simulink model "IMfault"  (R2017a)
settings: Solver=FixedStepAuto  StartTime=0.0  StopTime=0.6  MaxStep=1e-4  RelTol=1e-3
libraries: powerlib x24, dspxfrm3 x3, dspspect3 x3
settings Model: Creator=saeed  LastModifiedBy=Lenovo

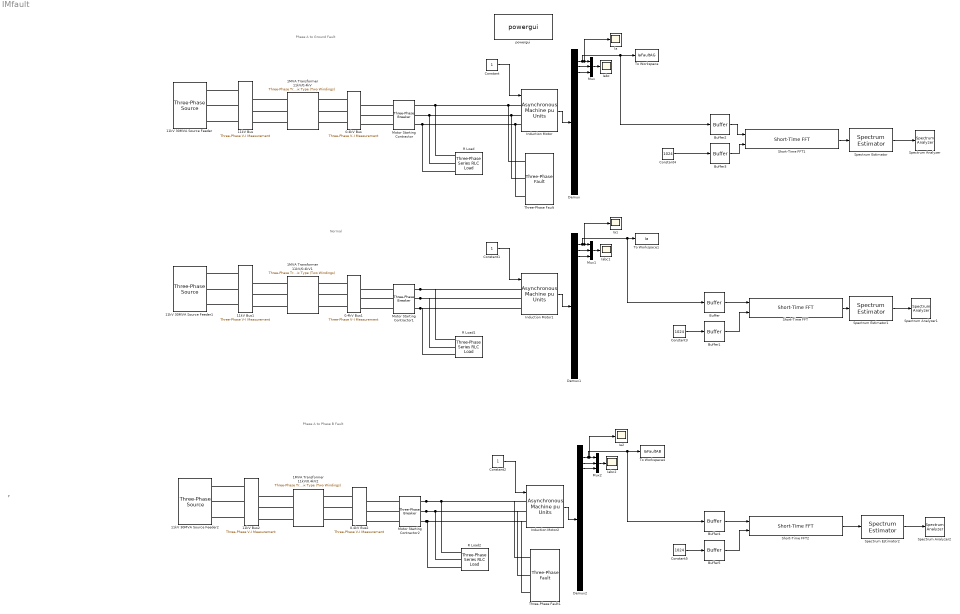
== system IMfault ==
  note: Normal
  note: P
  note: Phase A to Ground
      | Fault
  note: Phase A to Phase B
      | Fault
  0.4kV Bus : powerlib/Measurements/Three-Phase V-I Measurement  VoltageMeasurement=no  SetLabelV=off  LabelV=Vabc  Vpu=off  VpuLL=off  CurrentMeasurement=yes  SetLabelI=off  LabelI=Iabc  Ipu=off  Pbase=100e6  Vbase=500e3  OutputType=Complex  PhasorSimulation=off  PSBequivalent=0
  0.4kV Bus1 : powerlib/Measurements/Three-Phase V-I Measurement  VoltageMeasurement=no  SetLabelV=off  LabelV=Vabc  Vpu=off  VpuLL=off  CurrentMeasurement=yes  SetLabelI=off  LabelI=Iabc  Ipu=off  Pbase=100e6  Vbase=500e3  OutputType=Complex  PhasorSimulation=off  PSBequivalent=0
  0.4kV Bus2 : powerlib/Measurements/Three-Phase V-I Measurement  VoltageMeasurement=no  SetLabelV=off  LabelV=Vabc  Vpu=off  VpuLL=off  CurrentMeasurement=yes  SetLabelI=off  LabelI=Iabc  Ipu=off  Pbase=100e6  Vbase=500e3  OutputType=Complex  PhasorSimulation=off  PSBequivalent=0
  11kV Bus : powerlib/Measurements/Three-Phase V-I Measurement  VoltageMeasurement=no  SetLabelV=off  LabelV=Vabc  Vpu=off  VpuLL=off  CurrentMeasurement=yes  SetLabelI=off  LabelI=Iabc  Ipu=off  Pbase=100e6  Vbase=500e3  OutputType=Complex  PhasorSimulation=off  PSBequivalent=0
  11kV Bus1 : powerlib/Measurements/Three-Phase V-I Measurement  VoltageMeasurement=no  SetLabelV=off  LabelV=Vabc  Vpu=off  VpuLL=off  CurrentMeasurement=yes  SetLabelI=off  LabelI=Iabc  Ipu=off  Pbase=100e6  Vbase=500e3  OutputType=Complex  PhasorSimulation=off  PSBequivalent=0
  11kV Bus2 : powerlib/Measurements/Three-Phase V-I Measurement  VoltageMeasurement=no  SetLabelV=off  LabelV=Vabc  Vpu=off  VpuLL=off  CurrentMeasurement=yes  SetLabelI=off  LabelI=Iabc  Ipu=off  Pbase=100e6  Vbase=500e3  OutputType=Complex  PhasorSimulation=off  PSBequivalent=0
  11kV 30MVA Source Feeder : powerlib/Electrical Sources/Three-Phase Source  InternalConnection=Yg  VoltagePhases=off  Voltage=25e3  PhaseAngle=0  Voltage_phases=[25e3 25e3 25e3]/sqrt(3)  PhaseAngles_phases=[0 -120 +120]  Frequency=50  NonIdealSource=on  SpecifyImpedance=off  Resistance=0.8929  Inductance=16.58e-3  ShortCircuitLevel=100e6  BaseVoltage=25e3  XRratio=7  BusType=swing  Pref=10e3  Qref=0  Prefabc=[10e3, 10e3, 10e3]  Qrefabc=[0, 0, 0]  Qmin=-inf  Qmax=inf
  11kV 30MVA Source Feeder1 : powerlib/Electrical Sources/Three-Phase Source  InternalConnection=Yg  VoltagePhases=off  Voltage=25e3  PhaseAngle=0  Voltage_phases=[25e3 25e3 25e3]/sqrt(3)  PhaseAngles_phases=[0 -120 +120]  Frequency=50  NonIdealSource=on  SpecifyImpedance=off  Resistance=0.8929  Inductance=16.58e-3  ShortCircuitLevel=100e6  BaseVoltage=25e3  XRratio=7  BusType=swing  Pref=10e3  Qref=0  Prefabc=[10e3, 10e3, 10e3]  Qrefabc=[0, 0, 0]  Qmin=-inf  Qmax=inf
  11kV 30MVA Source Feeder2 : powerlib/Electrical Sources/Three-Phase Source  InternalConnection=Yg  VoltagePhases=off  Voltage=25e3  PhaseAngle=0  Voltage_phases=[25e3 25e3 25e3]/sqrt(3)  PhaseAngles_phases=[0 -120 +120]  Frequency=50  NonIdealSource=on  SpecifyImpedance=off  Resistance=0.8929  Inductance=16.58e-3  ShortCircuitLevel=100e6  BaseVoltage=25e3  XRratio=7  BusType=swing  Pref=10e3  Qref=0  Prefabc=[10e3, 10e3, 10e3]  Qrefabc=[0, 0, 0]  Qmin=-inf  Qmax=inf
  1MVA Transformer 11kV/0.4kV : powerlib/Elements/Three-Phase Transformer Inductance Matrix Type (Two Windings)  CoreType=Three-limb or five-limb core  Winding1Connection=Yg  Winding2Connection=Yg  AutoTransformer=on  Measurements=None  NominalPower=[100e3, 50]  VLLnom=[2400, 600]  WindingResistances=[0.01, 0.01]  NoLoadIexcPos=2  NoLoadPlossPos=1000  ShortCircuitReactancePos=0.06  ShortCircuitReactancePosAuto=0.06  NoLoadIexcZero=100  NoLoadPlossZero=1500  ShortCircuitReactanceZero=0.03  ShortCircuitReactanceZeroAuto=0.03
      settings: SourceProductName=Simscape Power Systems  SourceProductBaseCode=PS
  1MVA Transformer 11kV/0.4kV1 : powerlib/Elements/Three-Phase Transformer Inductance Matrix Type (Two Windings)  CoreType=Three-limb or five-limb core  Winding1Connection=Yg  Winding2Connection=Yg  AutoTransformer=on  Measurements=None  NominalPower=[100e3, 50]  VLLnom=[2400, 600]  WindingResistances=[0.01, 0.01]  NoLoadIexcPos=2  NoLoadPlossPos=1000  ShortCircuitReactancePos=0.06  ShortCircuitReactancePosAuto=0.06  NoLoadIexcZero=100  NoLoadPlossZero=1500  ShortCircuitReactanceZero=0.03  ShortCircuitReactanceZeroAuto=0.03
      settings: SourceProductName=Simscape Power Systems  SourceProductBaseCode=PS
  1MVA Transformer 11kV/0.4kV2 : powerlib/Elements/Three-Phase Transformer Inductance Matrix Type (Two Windings)  CoreType=Three-limb or five-limb core  Winding1Connection=Yg  Winding2Connection=Yg  AutoTransformer=on  Measurements=None  NominalPower=[100e3, 50]  VLLnom=[2400, 600]  WindingResistances=[0.01, 0.01]  NoLoadIexcPos=2  NoLoadPlossPos=1000  ShortCircuitReactancePos=0.06  ShortCircuitReactancePosAuto=0.06  NoLoadIexcZero=100  NoLoadPlossZero=1500  ShortCircuitReactanceZero=0.03  ShortCircuitReactanceZeroAuto=0.03
      settings: SourceProductName=Simscape Power Systems  SourceProductBaseCode=PS
  Buffer{,1..5} (6 alike) : Buffer  N=512  OutputFrames=off
  Constant : Constant
  Constant1 : Constant
  Constant2 : Constant
  Constant3 : Constant  Value=1024
  Constant4 : Constant  Value=1024
  Constant5 : Constant  Value=1024
  Demux : Demux  Outputs=22
  Demux1 : Demux  Outputs=22
  Demux2 : Demux  Outputs=22
  Ia : Scope
  Ia1 : Scope
  Ia2 : Scope
  Iabc : Scope
  Iabc1 : Scope
  Iabc2 : Scope
  Induction Motor : powerlib/Machines/Asynchronous Machine pu Units  RotorType=Squirrel-cage  PresetModel=No  MechanicalLoad=Speed w  ShowDetailedParameters=on  ReferenceFrame=Rotor  Units=pu  MeasurementBus=on  NominalParameters=[3730 460 50]  Stator=[0.01965 0.0397]  Rotor=[0.01909 0.0397]  Cage1=[0.01909 0.0397]  Cage2=[0.01909 0.0397]  Lm=1.354  Mechanical=[0.09526 0.05479 2]  PolePairs=2  InitialConditions="[ 1,0   0,0,0   0,0,0 ]"  SimulateSaturation=off  Saturation="[0.212,0.4201,0.8125,1.0979,1.4799,2.2457,3.2586,4.5763,6.4763 ;   0.5,0.7,0.9,1,1.1,1.2 ,1.3,1.4,1.5]"  LoadFlowParameters=0  TsPowergui=0  TsBlock=-1  IterativeModel=Trapezoidal non iterative  IterativeDiscreteModel=Trapezoidal non iterative  Pmec=0
      settings: SourceProductName=Simscape Power Systems  SourceProductBaseCode=PS
  Induction Motor1 : powerlib/Machines/Asynchronous Machine pu Units  RotorType=Squirrel-cage  PresetModel=No  MechanicalLoad=Speed w  ShowDetailedParameters=on  ReferenceFrame=Rotor  Units=pu  MeasurementBus=on  NominalParameters=[3730 460 50]  Stator=[0.01965 0.0397]  Rotor=[0.01909 0.0397]  Cage1=[0.01909 0.0397]  Cage2=[0.01909 0.0397]  Lm=1.354  Mechanical=[0.09526 0.05479 2]  PolePairs=2  InitialConditions="[ 1,0   0,0,0   0,0,0 ]"  SimulateSaturation=off  Saturation="[0.212,0.4201,0.8125,1.0979,1.4799,2.2457,3.2586,4.5763,6.4763 ;   0.5,0.7,0.9,1,1.1,1.2 ,1.3,1.4,1.5]"  LoadFlowParameters=0  TsPowergui=0  TsBlock=-1  IterativeModel=Trapezoidal non iterative  IterativeDiscreteModel=Trapezoidal non iterative  Pmec=0
      settings: SourceProductName=Simscape Power Systems  SourceProductBaseCode=PS
  Induction Motor2 : powerlib/Machines/Asynchronous Machine pu Units  RotorType=Squirrel-cage  PresetModel=No  MechanicalLoad=Speed w  ShowDetailedParameters=on  ReferenceFrame=Rotor  Units=pu  MeasurementBus=on  NominalParameters=[3730 460 50]  Stator=[0.01965 0.0397]  Rotor=[0.01909 0.0397]  Cage1=[0.01909 0.0397]  Cage2=[0.01909 0.0397]  Lm=1.354  Mechanical=[0.09526 0.05479 2]  PolePairs=2  InitialConditions="[ 1,0   0,0,0   0,0,0 ]"  SimulateSaturation=off  Saturation="[0.212,0.4201,0.8125,1.0979,1.4799,2.2457,3.2586,4.5763,6.4763 ;   0.5,0.7,0.9,1,1.1,1.2 ,1.3,1.4,1.5]"  LoadFlowParameters=0  TsPowergui=0  TsBlock=-1  IterativeModel=Trapezoidal non iterative  IterativeDiscreteModel=Trapezoidal non iterative  Pmec=0
      settings: SourceProductName=Simscape Power Systems  SourceProductBaseCode=PS
  Motor Starting Contractor : powerlib/Elements/Three-Phase Breaker  InitialState=open  SwitchA=on  SwitchB=on  SwitchC=on  SwitchTimes=[0.005]  External=off  BreakerResistance=0.01  SnubberResistance=1e6  SnubberCapacitance=inf  Measurements=None
  Motor Starting Contractor1 : powerlib/Elements/Three-Phase Breaker  InitialState=open  SwitchA=on  SwitchB=on  SwitchC=on  SwitchTimes=[0.005]  External=off  BreakerResistance=0.01  SnubberResistance=1e6  SnubberCapacitance=inf  Measurements=None
  Motor Starting Contractor2 : powerlib/Elements/Three-Phase Breaker  InitialState=open  SwitchA=on  SwitchB=on  SwitchC=on  SwitchTimes=[0.005]  External=off  BreakerResistance=0.01  SnubberResistance=1e6  SnubberCapacitance=inf  Measurements=None
  Mux : Mux  Inputs=3
  Mux1 : Mux  Inputs=3
  Mux2 : Mux  Inputs=3
  R Load : powerlib/Elements/Three-Phase Series RLC Load  LConnTagsString=A|B|C  Configuration=Y (grounded)  NominalVoltage=1000  Vabc=[1e3 1e3 1e3]  Vabcp=[1e3 1e3 1e3]  NominalFrequency=50  UnbalancedPower=off  ActivePower=10e3  InductivePower=100  CapacitivePower=100  Pabc=[10e3 9e3 11e3]  QLabc=[100 90 110]  QCabc=[100 90 110]  Pabcp=[10e3 9e3 11e3]  QLabcp=[100 90 110]  QCabcp=[100 90 110]  Measurements=None  LoadType=constant I
  R Load1 : powerlib/Elements/Three-Phase Series RLC Load  LConnTagsString=A|B|C  Configuration=Y (grounded)  NominalVoltage=1000  Vabc=[1e3 1e3 1e3]  Vabcp=[1e3 1e3 1e3]  NominalFrequency=60  UnbalancedPower=off  ActivePower=10e3  InductivePower=100  CapacitivePower=100  Pabc=[10e3 9e3 11e3]  QLabc=[100 90 110]  QCabc=[100 90 110]  Pabcp=[10e3 9e3 11e3]  QLabcp=[100 90 110]  QCabcp=[100 90 110]  Measurements=None  LoadType=constant I
  R Load2 : powerlib/Elements/Three-Phase Series RLC Load  LConnTagsString=A|B|C  Configuration=Y (grounded)  NominalVoltage=1000  Vabc=[1e3 1e3 1e3]  Vabcp=[1e3 1e3 1e3]  NominalFrequency=50  UnbalancedPower=off  ActivePower=10e3  InductivePower=100  CapacitivePower=100  Pabc=[10e3 9e3 11e3]  QLabc=[100 90 110]  QCabc=[100 90 110]  Pabcp=[10e3 9e3 11e3]  QLabcp=[100 90 110]  QCabcp=[100 90 110]  Measurements=None  LoadType=constant I
  Short-Time FFT : dspxfrm3/Short-Time FFT  W=512  OvLap=256  M=1024
      settings: SourceProductName=DSP System Toolbox  SourceProductBaseCode=DS
  Short-Time FFT1 : dspxfrm3/Short-Time FFT  W=512  OvLap=216  M=1024
      settings: SourceProductName=DSP System Toolbox  SourceProductBaseCode=DS
  Short-Time FFT2 : dspxfrm3/Short-Time FFT  W=512  OvLap=256  M=1024
      settings: SourceProductName=DSP System Toolbox  SourceProductBaseCode=DS
  Spectrum Analyzer : SpectrumAnalyzer
  Spectrum Analyzer1 : SpectrumAnalyzer
  Spectrum Analyzer2 : SpectrumAnalyzer
  Spectrum Estimator : dspspect3/Spectrum Estimator  Method=Filter bank  NumTapsPerBand=12  SpectrumType=Power density  FrequencyResolutionMethod=Auto  FilterBankResolutionMethod=Auto  RBW=5  WindowLength=1024  FrequencyBandsSource=Same as input frame size  FrequencyBands=1024  FFTLengthSource=Auto  FFTLength=1024  InheritSampleRate=on  SampleRate=44100  Window=Hann  SidelobeAttenuation=60  SpectralAverages=1  Overlap=0  ReferenceLoad=1  FrequencyRange=Centered  PowerUnits=dBm  OutputMaxHoldSpectrum=off  OutputMinHoldSpectrum=off  OutputFrequencyVector=off  OutputRBW=off  SimulateUsing=Code generation
      settings: SourceProductName=DSP System Toolbox  SourceProductBaseCode=DS
  Spectrum Estimator1 : dspspect3/Spectrum Estimator  Method=Filter bank  NumTapsPerBand=12  SpectrumType=Power  FrequencyResolutionMethod=Auto  FilterBankResolutionMethod=Auto  RBW=5  WindowLength=1024  FrequencyBandsSource=Same as input frame size  FrequencyBands=1024  FFTLengthSource=Auto  FFTLength=1024  InheritSampleRate=on  SampleRate=44100  Window=Hann  SidelobeAttenuation=60  SpectralAverages=1  Overlap=0  ReferenceLoad=1  FrequencyRange=Centered  PowerUnits=dBm  OutputMaxHoldSpectrum=off  OutputMinHoldSpectrum=off  OutputFrequencyVector=off  OutputRBW=off  SimulateUsing=Code generation
      settings: SourceProductName=DSP System Toolbox  SourceProductBaseCode=DS
  Spectrum Estimator2 : dspspect3/Spectrum Estimator  Method=Filter bank  NumTapsPerBand=12  SpectrumType=Power  FrequencyResolutionMethod=Auto  FilterBankResolutionMethod=Auto  RBW=5  WindowLength=1024  FrequencyBandsSource=Same as input frame size  FrequencyBands=1024  FFTLengthSource=Auto  FFTLength=1024  InheritSampleRate=on  SampleRate=44100  Window=Hann  SidelobeAttenuation=60  SpectralAverages=1  Overlap=0  ReferenceLoad=1  FrequencyRange=Centered  PowerUnits=dBm  OutputMaxHoldSpectrum=off  OutputMinHoldSpectrum=off  OutputFrequencyVector=off  OutputRBW=off  SimulateUsing=Code generation
      settings: SourceProductName=DSP System Toolbox  SourceProductBaseCode=DS
  Three-Phase Fault : powerlib/Elements/Three-Phase Fault  InitialStates=1  FaultA=on  FaultB=off  FaultC=off  GroundFault=on  SwitchTimes=[0.3 0.6]  External=off  SwitchStatus=NaN  FaultResistance=0.001  GroundResistance=0.01  SnubberResistance=1e6  SnubberCapacitance=inf  Measurements=Fault currents
  Three-Phase Fault1 : powerlib/Elements/Three-Phase Fault  InitialStates=1  FaultA=on  FaultB=on  FaultC=off  GroundFault=off  SwitchTimes=[0.3 0.6]  External=off  SwitchStatus=NaN  FaultResistance=0.001  GroundResistance=0.01  SnubberResistance=1e6  SnubberCapacitance=inf  Measurements=Fault currents
  To Workspace : ToWorkspace  VariableName=IaFaultAG  SaveFormat=Structure With Time  SampleTime=-1
  To Workspace1 : ToWorkspace  VariableName=Ia  SaveFormat=Structure With Time  SampleTime=-1
  To Workspace4 : ToWorkspace  VariableName=IaFaultAB  SaveFormat=Structure With Time  SampleTime=-1
  powergui : powerlib/powergui  Priority=1  SimulationMode=Discrete  SampleTime=50e-6  frequency=60  Iterations=50  frequencyindice=50  Pbase=100e6  ErrMax=1e-4  UnitsV=kV  UnitsW=MW  buscounter=0  FunctionMessages=off  echomessages=off  EnableUseOfTLC=off  CurrentSourceSwitches=off  DisableSnubberDevices=off  DisableRonSwitches=off  DisableVfSwitches=off  DisplayEquations=off  SolverType=Tustin/Backward Euler (TBE)  Interpol=off  ExternalGateDelay=off  methode=off  Ts=100  x0status=blocks  SPID=off  SwTol=0  HookPort=off  RestoreLinks=warning  ResistiveCurrentMeasurement=off  Frange=[0:2:500]  Ylog=off  Xlog=on  ShowGrid=off  save=off  variable=ZData  structure=Ia  ZoomFFT=off  StartTime=0.0  cycles=25  DisplayStyle=1  fundamental=50  FreqAxis=off  MaxFrequency=300  frequencyindicesteady=1  RmsSteady=1  display=off
  wires:
  Constant/1 -> Induction Motor/1
  Induction Motor/1 -> Demux/1
  Demux/2 -> Mux/2
  Demux/3 -> Mux/3
  Mux/1 -> Iabc/1
  Demux1/2 -> Mux1/2
  Demux1/3 -> Mux1/3
  Induction Motor1/1 -> Demux1/1
  Demux1/1 -> Buffer/1, To Workspace1/1, Ia1/1, Mux1/1
  Mux1/1 -> Iabc1/1
  Constant1/1 -> Induction Motor1/1
  Mux2/1 -> Iabc2/1
  Induction Motor2/1 -> Demux2/1
  Demux2/3 -> Mux2/3
  Demux2/2 -> Mux2/2
  Constant2/1 -> Induction Motor2/1
  Short-Time FFT/1 -> Spectrum Estimator1/1
  Buffer/1 -> Short-Time FFT/1
  Constant3/1 -> Buffer1/1
  Buffer1/1 -> Short-Time FFT/2
  Buffer3/1 -> Short-Time FFT1/2
  Demux/1 -> Buffer2/1, To Workspace/1, Ia/1, Mux/1
  Short-Time FFT1/1 -> Spectrum Estimator/1
  Buffer2/1 -> Short-Time FFT1/1
  Buffer5/1 -> Short-Time FFT2/2
  Demux2/1 -> Buffer4/1, To Workspace4/1, Ia2/1, Mux2/1
  Short-Time FFT2/1 -> Spectrum Estimator2/1
  Buffer4/1 -> Short-Time FFT2/1
  Constant5/1 -> Buffer5/1
  Constant4/1 -> Buffer3/1
  Spectrum Estimator1/1 -> Spectrum Analyzer1/1
  Spectrum Estimator/1 -> Spectrum Analyzer/1
  Spectrum Estimator2/1 -> Spectrum Analyzer2/1
  connections:
  11kV Bus/LConn1 -- 11kV 30MVA Source Feeder/RConn1
  11kV Bus/LConn2 -- 11kV 30MVA Source Feeder/RConn2
  11kV Bus/LConn3 -- 11kV 30MVA Source Feeder/RConn3
  1MVA Transformer 11kV/0.4kV/LConn1 -- 11kV Bus/RConn1
  1MVA Transformer 11kV/0.4kV/LConn2 -- 11kV Bus/RConn2
  1MVA Transformer 11kV/0.4kV/LConn3 -- 11kV Bus/RConn3
  0.4kV Bus/LConn2 -- 1MVA Transformer 11kV/0.4kV/RConn2
  0.4kV Bus/LConn1 -- 1MVA Transformer 11kV/0.4kV/RConn1
  0.4kV Bus/LConn3 -- 1MVA Transformer 11kV/0.4kV/RConn3
  Motor Starting Contractor/LConn1 -- 0.4kV Bus/RConn1
  Motor Starting Contractor/LConn2 -- 0.4kV Bus/RConn2
  Motor Starting Contractor/LConn3 -- 0.4kV Bus/RConn3
  Induction Motor/LConn1 -- Three-Phase Fault/LConn1 -- R Load/LConn1 -- Motor Starting Contractor/RConn1
  Induction Motor/LConn2 -- Three-Phase Fault/LConn2 -- R Load/LConn2 -- Motor Starting Contractor/RConn2
  Induction Motor/LConn3 -- Three-Phase Fault/LConn3 -- R Load/LConn3 -- Motor Starting Contractor/RConn3
  Motor Starting Contractor1/RConn2 -- Induction Motor1/LConn2 -- R Load1/LConn2
  Motor Starting Contractor1/RConn1 -- Induction Motor1/LConn1 -- R Load1/LConn1
  Motor Starting Contractor1/RConn3 -- Induction Motor1/LConn3 -- R Load1/LConn3
  0.4kV Bus1/LConn3 -- 1MVA Transformer 11kV/0.4kV1/RConn3
  Motor Starting Contractor1/LConn1 -- 0.4kV Bus1/RConn1
  1MVA Transformer 11kV/0.4kV1/LConn1 -- 11kV Bus1/RConn1
  Motor Starting Contractor1/LConn2 -- 0.4kV Bus1/RConn2
  0.4kV Bus1/LConn1 -- 1MVA Transformer 11kV/0.4kV1/RConn1
  11kV Bus1/LConn1 -- 11kV 30MVA Source Feeder1/RConn1
  Motor Starting Contractor1/LConn3 -- 0.4kV Bus1/RConn3
  0.4kV Bus1/LConn2 -- 1MVA Transformer 11kV/0.4kV1/RConn2
  1MVA Transformer 11kV/0.4kV1/LConn3 -- 11kV Bus1/RConn3
  11kV Bus1/LConn2 -- 11kV 30MVA Source Feeder1/RConn2
  1MVA Transformer 11kV/0.4kV1/LConn2 -- 11kV Bus1/RConn2
  11kV Bus1/LConn3 -- 11kV 30MVA Source Feeder1/RConn3
  Motor Starting Contractor2/RConn1 -- R Load2/LConn1 -- Induction Motor2/LConn1 -- Three-Phase Fault1/LConn1
  Motor Starting Contractor2/RConn3 -- R Load2/LConn3 -- Induction Motor2/LConn3 -- Three-Phase Fault1/LConn3
  Motor Starting Contractor2/RConn2 -- R Load2/LConn2 -- Induction Motor2/LConn2 -- Three-Phase Fault1/LConn2
  0.4kV Bus2/LConn1 -- 1MVA Transformer 11kV/0.4kV2/RConn1
  11kV Bus2/LConn2 -- 11kV 30MVA Source Feeder2/RConn2
  Motor Starting Contractor2/LConn1 -- 0.4kV Bus2/RConn1
  0.4kV Bus2/LConn2 -- 1MVA Transformer 11kV/0.4kV2/RConn2
  0.4kV Bus2/LConn3 -- 1MVA Transformer 11kV/0.4kV2/RConn3
  Motor Starting Contractor2/LConn3 -- 0.4kV Bus2/RConn3
  1MVA Transformer 11kV/0.4kV2/LConn1 -- 11kV Bus2/RConn1
  1MVA Transformer 11kV/0.4kV2/LConn2 -- 11kV Bus2/RConn2
  11kV Bus2/LConn1 -- 11kV 30MVA Source Feeder2/RConn1
  1MVA Transformer 11kV/0.4kV2/LConn3 -- 11kV Bus2/RConn3
  Motor Starting Contractor2/LConn2 -- 0.4kV Bus2/RConn2
  11kV Bus2/LConn3 -- 11kV 30MVA Source Feeder2/RConn3
